simulink model "ASSIG2_v5"  (R2020a)
settings: Solver=FixedStepAuto  StartTime=0.0  StopTime=10.0  FixedStep=1e-3  RelTol=1e-3  EnableMultiTasking=on
undefined symbols (not defined in the file): A0, A1, D0, D1, D10, D11, D12, D13, D2, D3, D4, D5, D6, D7, D8, D9, magnitude, PTA0, PTA1, PTA2, PTB2, PTB23, PTB3, PTB9, PTC16, PTC17, PTC2, PTC3, PTC4, PTD0, PTD1, PTD2, PTD3
libraries: etargetslib x21, frdmk64flib x20
settings Model: ExtModeTrigDuration=5  Creator=Nour  LastModifiedBy=Khaled
settings OptimizationCC: EnhancedBackFolding=on  PassReuseOutputArgsAs=Individual arguments  ZeroExternalMemoryAtStartup=off  ZeroInternalMemoryAtStartup=off  MaxStackSize=64  OptimizeBlockOrder=speed  DifferentSizesBufferReuse=on  OptimizationCustomize=off  EfficientTunableParamExpr=on
settings DebuggingCC: ParameterTunabilityLossMsg=error  UnderSpecifiedDimensionMsg=error
settings HardwareCC: ProdBitPerPointer=32  ProdBitPerSizeT=32  ProdBitPerPtrDiffT=32  ProdLargestAtomicInteger=Long  ProdLargestAtomicFloat=Double  ProdWordSize=32  ProdHWDeviceType=ARM Compatible->ARM Cortex
settings SFSimCC: MATLABDynamicMemAlloc=off
settings RTWCC: SystemTargetFile=ert.tlc  HardwareBoard=NXP FRDM-K64F  TemplateMakefile=ert_default_tmf  Toolchain=GNU Tools for ARM Embedded Processors
settings CodeAppCC: ForceParamTrailComments=on  IgnoreCustomStorageClasses=off  OperatorAnnotations=on  SimulinkDataObjDesc=on  SFDataObjDesc=on  InsertBlockDesc=on

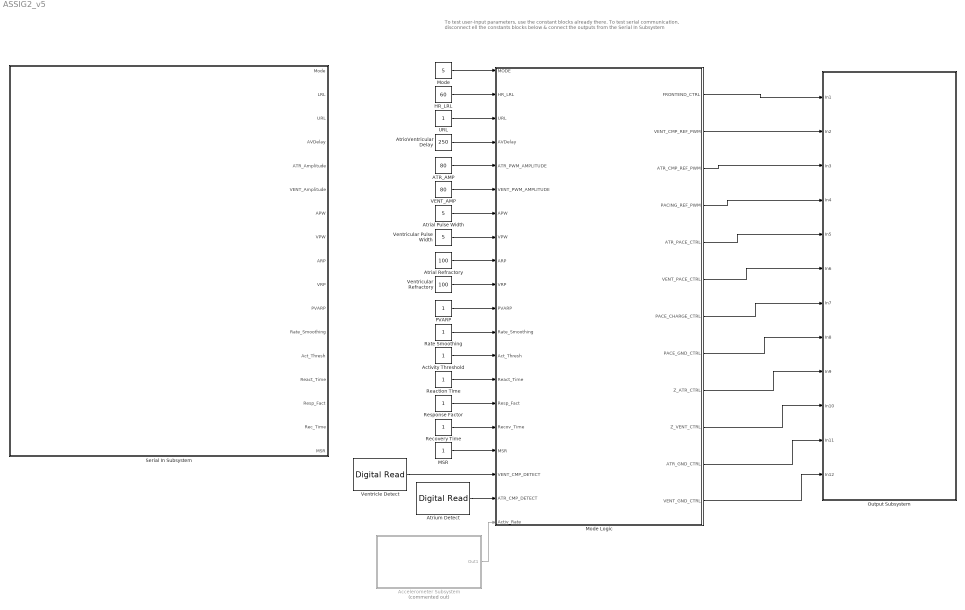
== system ASSIG2_v5 ==
  note: To test user-input parameters, use the constant blocks already there.
      | To test serial communication, disconnect ell the constants blocks below & connect the outputs from the Serial In Subsystem
  ATR_AMP : Constant  Value=80  OutDataTypeStr=uint8
  Accelerometer Subsystem : Subsystem  Commented=on
  Activity Threshold : Constant  OutDataTypeStr=single
  Atrial Pulse Width : Constant  Value=5  OutDataTypeStr=uint16
  Atrial Refractory : Constant  Value=100  OutDataTypeStr=uint16
  AtrioVentricular Delay : Constant  Value=250  OutDataTypeStr=uint16
  Atrium Detect : frdmk64flib/Digital Read  Whichpin=PTC16 (D0)  SampleTime=-1
  HR_LRL : Constant  Value=60  OutDataTypeStr=uint16
  MSR : Constant  OutDataTypeStr=uint16
  Mode : Constant  Value=5  OutDataTypeStr=uint8
  Mode Logic : Stateflow chart  TreatAsAtomicUnit=on
  Output Subsystem : Subsystem
  PVARP : Constant  OutDataTypeStr=uint16
  Rate Smoothing : Constant  OutDataTypeStr=uint8
  Reaction Time : Constant  OutDataTypeStr=uint16
  Recovery Time : Constant  OutDataTypeStr=uint16
  Response Factor : Constant  OutDataTypeStr=uint16
  Serial In Subsystem : Subsystem
  URL : Constant  OutDataTypeStr=uint8
  VENT_AMP : Constant  Value=80  OutDataTypeStr=uint8
  Ventricle Detect : frdmk64flib/Digital Read  Whichpin=PTC17 (D1)  SampleTime=-1
  Ventricular Pulse Width : Constant  Value=5  OutDataTypeStr=uint16
  Ventricular Refractory : Constant  Value=100  OutDataTypeStr=uint16
  wires:
  HR_LRL/1 -> Mode Logic/2(HR_LRL)
  Mode/1 -> Mode Logic/1(MODE)
  Atrial Refractory/1 -> Mode Logic/9(ARP)
  Ventricular Refractory/1 -> Mode Logic/10(VRP)
  Atrial Pulse Width/1 -> Mode Logic/7(APW)
  Ventricle Detect/1 -> Mode Logic/18(VENT_CMP_DETECT)
  Atrium Detect/1 -> Mode Logic/19(ATR_CMP_DETECT)
  Ventricular Pulse Width/1 -> Mode Logic/8(VPW)
  AtrioVentricular Delay/1 -> Mode Logic/4(AVDelay)
  MSR/1 -> Mode Logic/17(MSR)
  ATR_AMP/1 -> Mode Logic/5(ATR_PWM_AMPLITUDE)
  VENT_AMP/1 -> Mode Logic/6(VENT_PWM_AMPLITUDE)
  Mode Logic/1(FRONTEND_CTRL) -> Output Subsystem/1(In1)
  Mode Logic/2(VENT_CMP_REF_PWM) -> Output Subsystem/2(In2)
  Mode Logic/3(ATR_CMP_REF_PWM) -> Output Subsystem/3(In3)
  Mode Logic/4(PACING_REF_PWM) -> Output Subsystem/4(In4)
  Mode Logic/5(ATR_PACE_CTRL) -> Output Subsystem/5(In5)
  Mode Logic/6(VENT_PACE_CTRL) -> Output Subsystem/6(In6)
  Mode Logic/7(PACE_CHARGE_CTRL) -> Output Subsystem/7(In7)
  Mode Logic/8(PACE_GND_CTRL) -> Output Subsystem/8(In8)
  Mode Logic/9(Z_ATR_CTRL) -> Output Subsystem/9(In9)
  Mode Logic/10(Z_VENT_CTRL) -> Output Subsystem/10(In10)
  Mode Logic/11(ATR_GND_CTRL) -> Output Subsystem/11(In11)
  Mode Logic/12(VENT_GND_CTRL) -> Output Subsystem/12(In12)
  URL/1 -> Mode Logic/3(URL)
  PVARP/1 -> Mode Logic/11(PVARP)
  Recovery Time/1 -> Mode Logic/16(Recov_Time)
  Response Factor/1 -> Mode Logic/15(Resp_Fact)
  Reaction Time/1 -> Mode Logic/14(React_Time)
  Activity Threshold/1 -> Mode Logic/13(Act_Thresh)
  Rate Smoothing/1 -> Mode Logic/12(Rate_Smoothing)
  Accelerometer Subsystem/1(Out1) -> Mode Logic/20(Activ_Rate)

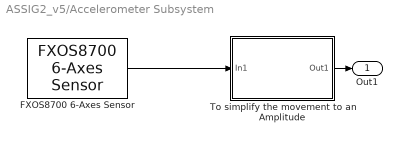
== system ASSIG2_v5/Accelerometer Subsystem ==
  FXOS8700 6-Axes Sensor : frdmk64flib/FXOS8700 6-Axes Sensor  Activesensor=Accelerometer only  ODR=800Hz  HybridODR=400Hz  Accelfullrange=-4g to +4g  SampleTime=-1
  To simplify the movement to an Amplitude : Subsystem
  Out1 : Outport
  wires:
  FXOS8700 6-Axes Sensor/1 -> To simplify the movement to an Amplitude/1(In1)
  To simplify the movement to an Amplitude/1(Out1) -> Out1/1

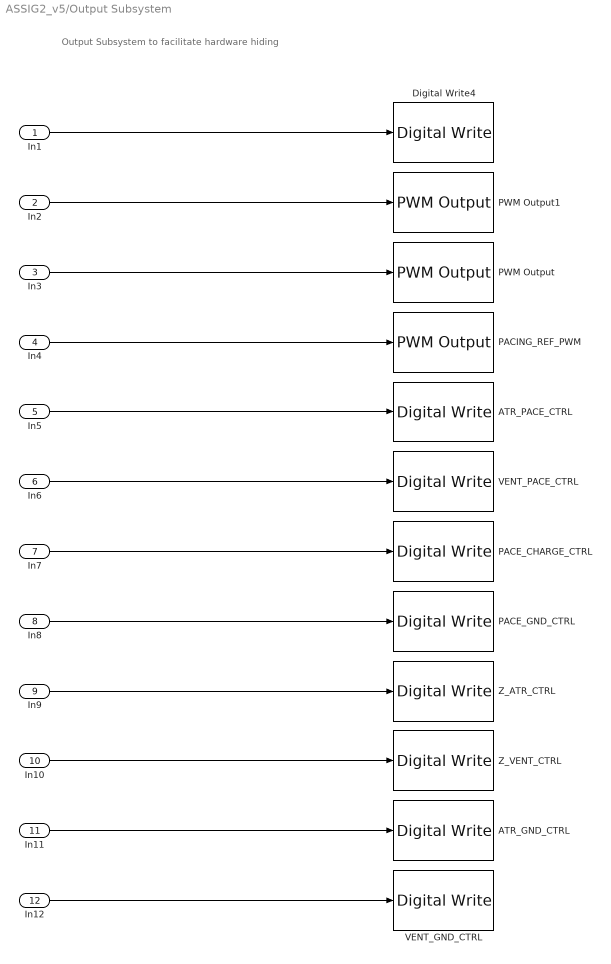
== system ASSIG2_v5/Output Subsystem ==
  note: Output Subsystem to facilitate hardware hiding
  In1 : Inport
  In2 : Inport  Port=2
  In3 : Inport  Port=3
  In4 : Inport  Port=4
  In5 : Inport  Port=5
  In6 : Inport  Port=6
  In7 : Inport  Port=7
  In8 : Inport  Port=8
  In9 : Inport  Port=9
  In10 : Inport  Port=10
  In11 : Inport  Port=11
  In12 : Inport  Port=12
  ATR_GND_CTRL : frdmk64flib/Digital Write  Whichpin=PTD2 (D11)
  ATR_PACE_CTRL : frdmk64flib/Digital Write  Whichpin=PTA0 (D8)
  Digital Write4 : frdmk64flib/Digital Write  Whichpin=PTD1 (D13)
  PACE_CHARGE_CTRL : frdmk64flib/Digital Write  Whichpin=PTB9 (D2)
  PACE_GND_CTRL : frdmk64flib/Digital Write  Whichpin=PTD0 (D10)
  PACING_REF_PWM : frdmk64flib/PWM Output  Whichpin=PTA2 (D5)  InitialFrequency=2000  InitialDutyCycle=80
  PWM Output : frdmk64flib/PWM Output  Whichpin=PTC2 (D6)  InitialFrequency=2000  InitialDutyCycle=20
  PWM Output1 : frdmk64flib/PWM Output  Whichpin=PTA1 (D3)  InitialFrequency=2000  InitialDutyCycle=20
  VENT_GND_CTRL : frdmk64flib/Digital Write  Whichpin=PTD3 (D12)
  VENT_PACE_CTRL : frdmk64flib/Digital Write  Whichpin=PTC4 (D9)
  Z_ATR_CTRL : frdmk64flib/Digital Write  Whichpin=PTB23 (D4)
  Z_VENT_CTRL : frdmk64flib/Digital Write  Whichpin=PTC3 (D7)
  wires:
  In7/1 -> PACE_CHARGE_CTRL/1
  In12/1 -> VENT_GND_CTRL/1
  In1/1 -> Digital Write4/1
  In4/1 -> PACING_REF_PWM/1
  In8/1 -> PACE_GND_CTRL/1
  In6/1 -> VENT_PACE_CTRL/1
  In9/1 -> Z_ATR_CTRL/1
  In10/1 -> Z_VENT_CTRL/1
  In11/1 -> ATR_GND_CTRL/1
  In2/1 -> PWM Output1/1
  In5/1 -> ATR_PACE_CTRL/1
  In3/1 -> PWM Output/1

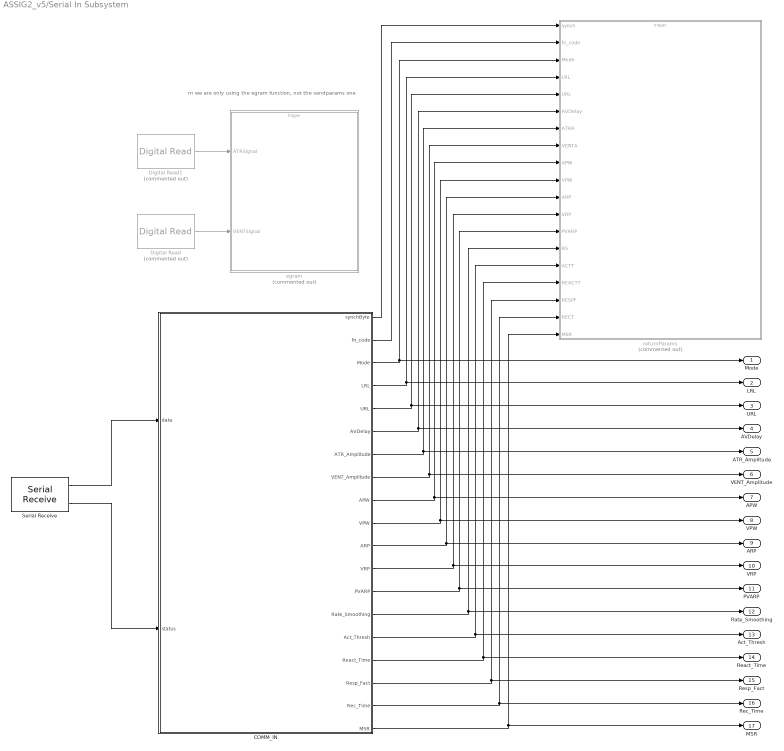
== system ASSIG2_v5/Serial In Subsystem ==
  note: rn we are only using the egram function, not the sendparams one
  COMM_IN : Stateflow chart  TreatAsAtomicUnit=on
  Digital Read : frdmk64flib/Digital Read  Commented=on  Whichpin=PTB3 (A1)  SampleTime=-1
  Digital Read1 : frdmk64flib/Digital Read  Commented=on  Whichpin=PTB2 (A0)  SampleTime=-1
  Serial Receive : frdmk64flib/Serial Receive  SCIModule=0  Baudrate=uint32(9600)  Parity=None  StopBits=1  HardwareFlowControl=None  ByteOrder=LittleEndian  DataType=uint8  DataLength=26  BlockingMode=off  OutputStatus=on  SampleTime=-1
  egram : Subsystem  Commented=on
  returnParams : Subsystem  Commented=on
  Mode : Outport
  LRL : Outport  Port=2
  URL : Outport  Port=3
  AVDelay : Outport  Port=4
  ATR_Amplitude : Outport  Port=5
  VENT_Amplitude : Outport  Port=6
  APW : Outport  Port=7
  VPW : Outport  Port=8
  ARP : Outport  Port=9
  VRP : Outport  Port=10
  PVARP : Outport  Port=11
  Rate_Smoothing : Outport  Port=12
  Act_Thresh : Outport  Port=13
  React_Time : Outport  Port=14
  Resp_Fact : Outport  Port=15
  Rec_Time : Outport  Port=16
  MSR : Outport  Port=17
  wires:
  COMM_IN/5(URL) -> returnParams/5(URL), URL/1
  COMM_IN/11(ARP) -> returnParams/11(ARP), ARP/1
  COMM_IN/6(AVDelay) -> returnParams/6(AVDelay), AVDelay/1
  Serial Receive/1 -> COMM_IN/1(data)
  COMM_IN/4(LRL) -> returnParams/4(LRL), LRL/1
  COMM_IN/10(VPW) -> returnParams/10(VPW), VPW/1
  Serial Receive/2 -> COMM_IN/2(status)
  COMM_IN/8(VENT_Amplitude) -> returnParams/8(VENTA), VENT_Amplitude/1
  COMM_IN/7(ATR_Amplitude) -> returnParams/7(ATRA), ATR_Amplitude/1
  COMM_IN/17(Resp_Fact) -> returnParams/17(RESPF), Resp_Fact/1
  COMM_IN/3(Mode) -> Mode/1, returnParams/3(Mode)
  COMM_IN/14(Rate_Smoothing) -> returnParams/14(RS), Rate_Smoothing/1
  COMM_IN/16(React_Time) -> returnParams/16(REACTT), React_Time/1
  COMM_IN/12(VRP) -> returnParams/12(VRP), VRP/1
  COMM_IN/9(APW) -> returnParams/9(APW), APW/1
  COMM_IN/18(Rec_Time) -> returnParams/18(RECT), Rec_Time/1
  COMM_IN/19(MSR) -> returnParams/19(MSR), MSR/1
  COMM_IN/15(Act_Thresh) -> returnParams/15(ACTT), Act_Thresh/1
  COMM_IN/13(PVARP) -> returnParams/13(PVARP), PVARP/1
  Digital Read1/1 -> egram/1(ATRSignal)
  Digital Read/1 -> egram/2(VENTSignal)
  COMM_IN/1(synchByte) -> returnParams/1(synch)
  COMM_IN/2(fn_code) -> returnParams/2(fn_code)

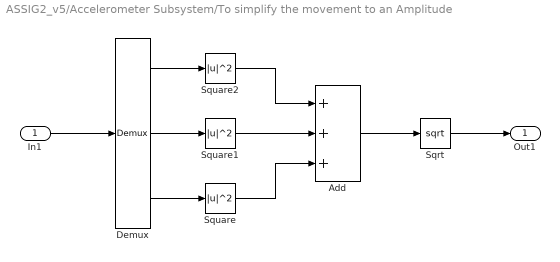
== system ASSIG2_v5/Accelerometer Subsystem/To simplify the movement to an Amplitude ==
  In1 : Inport
  Add : Sum  Inputs=+++
  Demux : Demux  Outputs=3
  Sqrt : Sqrt  OutputSignalType=real  OutDataTypeStr=single  IntermediateResultsDataTypeStr=double  SaturateOnIntegerOverflow=on
  Square : Math  Operator=magnitude^2  OutDataTypeStr=double  SaturateOnIntegerOverflow=on
  Square1 : Math  Operator=magnitude^2  OutDataTypeStr=double  SaturateOnIntegerOverflow=on
  Square2 : Math  Operator=magnitude^2  OutDataTypeStr=double  SaturateOnIntegerOverflow=on
  Out1 : Outport
  wires:
  In1/1 -> Demux/1
  Demux/3 -> Square/1
  Demux/2 -> Square1/1
  Demux/1 -> Square2/1
  Square2/1 -> Add/1
  Square1/1 -> Add/2
  Square/1 -> Add/3
  Add/1 -> Sqrt/1
  Sqrt/1 -> Out1/1

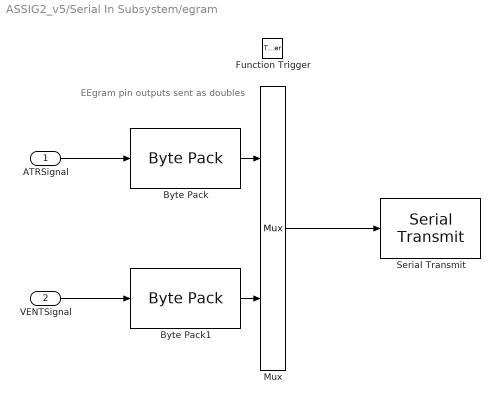
== system ASSIG2_v5/Serial In Subsystem/egram ==
  note: EEgram pin outputs sent as doubles
  ATRSignal : Inport
  VENTSignal : Inport  Port=2
  Function Trigger : TriggerPort  TriggerType=function-call  IsSimulinkFunction=on  FunctionName=eegram  VariantControl=Variant  PortDimensions=1
  Byte Pack : etargetslib/Byte Pack  datatypes={'double'}  byteAlign=1
  Byte Pack1 : etargetslib/Byte Pack  datatypes={'double'}  byteAlign=1
  Mux : Mux  Inputs=2
  Serial Transmit : frdmk64flib/Serial Transmit  SCIModule=0  Baudrate=uint32(9600)  Parity=None  StopBits=1  HardwareFlowControl=None  ByteOrder=LittleEndian  BlockingMode=on  OutputStatus=off
  wires:
  ATRSignal/1 -> Byte Pack/1
  Byte Pack1/1 -> Mux/2
  Byte Pack/1 -> Mux/1
  VENTSignal/1 -> Byte Pack1/1
  Mux/1 -> Serial Transmit/1

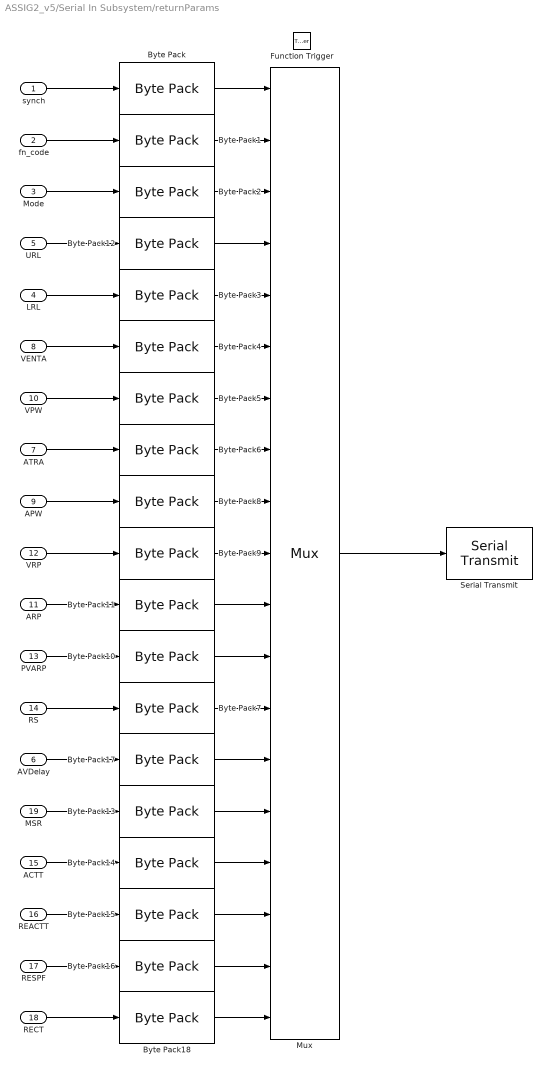
== system ASSIG2_v5/Serial In Subsystem/returnParams ==
  synch : Inport
  fn_code : Inport  Port=2
  Mode : Inport  Port=3
  LRL : Inport  Port=4
  URL : Inport  Port=5
  AVDelay : Inport  Port=6
  ATRA : Inport  Port=7
  VENTA : Inport  Port=8
  APW : Inport  Port=9
  VPW : Inport  Port=10
  ARP : Inport  Port=11
  VRP : Inport  Port=12
  PVARP : Inport  Port=13
  RS : Inport  Port=14
  ACTT : Inport  Port=15
  REACTT : Inport  Port=16
  RESPF : Inport  Port=17
  RECT : Inport  Port=18
  MSR : Inport  Port=19
  Function Trigger : TriggerPort  TriggerType=function-call  IsSimulinkFunction=on  FunctionName=returnParams  VariantControl=Variant  PortDimensions=1
  Byte Pack{,1..8,12..16,18} (15 alike) : etargetslib/Byte Pack  datatypes={'uint8'}  byteAlign=1
  Byte Pack{9..11,17} (4 alike) : etargetslib/Byte Pack  datatypes={'uint16'}  byteAlign=1
  Mux : Mux  Inputs=19
  Serial Transmit : frdmk64flib/Serial Transmit  SCIModule=0  Baudrate=uint32(9600)  Parity=None  StopBits=1  HardwareFlowControl=None  ByteOrder=LittleEndian  BlockingMode=on  OutputStatus=off
  wires:
  Byte Pack1/1 -> Mux/2
  Byte Pack/1 -> Mux/1
  Mux/1 -> Serial Transmit/1
  Byte Pack6/1 -> Mux/8
  Byte Pack2/1 -> Mux/3
  Byte Pack12/1 -> Mux/4
  Byte Pack3/1 -> Mux/5
  Byte Pack4/1 -> Mux/6
  Byte Pack5/1 -> Mux/7
  Byte Pack8/1 -> Mux/9
  Byte Pack11/1 -> Mux/11
  Byte Pack9/1 -> Mux/10
  Byte Pack10/1 -> Mux/12
  Byte Pack7/1 -> Mux/13
  Byte Pack16/1 -> Mux/18
  Byte Pack15/1 -> Mux/17
  Byte Pack14/1 -> Mux/16
  Byte Pack13/1 -> Mux/15
  Byte Pack17/1 -> Mux/14
  fn_code/1 -> Byte Pack1/1
  synch/1 -> Byte Pack/1
  Mode/1 -> Byte Pack2/1
  URL/1 -> Byte Pack12/1
  LRL/1 -> Byte Pack3/1
  VENTA/1 -> Byte Pack4/1
  VPW/1 -> Byte Pack5/1
  ATRA/1 -> Byte Pack6/1
  APW/1 -> Byte Pack8/1
  VRP/1 -> Byte Pack9/1
  ARP/1 -> Byte Pack11/1
  PVARP/1 -> Byte Pack10/1
  RS/1 -> Byte Pack7/1
  AVDelay/1 -> Byte Pack17/1
  MSR/1 -> Byte Pack13/1
  ACTT/1 -> Byte Pack14/1
  REACTT/1 -> Byte Pack15/1
  RESPF/1 -> Byte Pack16/1
  RECT/1 -> Byte Pack18/1
  Byte Pack18/1 -> Mux/19

== stateflow chart ASSIG2_v5/Serial In Subsystem/COMM_IN ==
  state SET_PARAM
    %% initial typecast of values through
    %% serial communication
    Mode = typecast(data(3), 'uint8');
    URL = typecast(data(4), 'uint8');
    LRL_t = typecast(data(5), 'uint8');
    VENT_Amplitude = typecast(data(6), 'uint8');
    VPW_t = typecast(data(7), 'uint8');
    ATR_Amplitude = typecast(data(8), 'uint8');
    APW_t = typecast(data(9), 'uint8');
    VRP = typecast(data(10:11), 'uint16');
    ARP = typecast(data(12:13), 'uint16');
    PVARP = typecast(data(14:15), 'uint16');
    Rate_Smoothing = typecast(data(16), 'uint8');
    AVDelay = typecast(data(17: 18), 'uint16');
    MSR_t = typecast(data(19), 'uint8');
    Act_Thresh = typecast(data(20:23), 'single');
    React_t = typecast(data(24), 'uint8');
    Resp_t = typecast(data(25), 'uint8');
    Rec_t = typecast(data(26), 'uint8');
    %% 2ndary typecast
    LRL  = uint16(LRL_t);
    VPW  = uint16(VPW_t);
    APW  = uint16(APW_t);
    MSR  = uint16(MSR_t);
    React_Time = uint16(React_t);
    Resp_Fact = uint16(Resp_t);
    Rec_Time = uint16(Rec_t);
  state INITIAL
    %% Setting initial, default values of parameters
    entry:
    Mode = 0;
    URL = 0;
    LRL = 0;
    VENT_Amplitude = 0;
    VPW = 0;
    ATR_Amplitude = 0;
    APW = 0;
    VRP = 0;
    ARP = 0;
    PVARP = 0;
    Rate_Smoothing = 0;
    AVDelay = 0;
    MSR = 0;
    Act_Thresh = 0;
    React_Time = 0;
    Resp_Fact = 0;
    Rec_Time = 0;
  state STANDBY
    %% Waiting for COM
    %% function code values;
    %% 55 -> set params
    %% 22 -> eegram
    %% 33 -> return params
    synchByte = typecast(data(1), 'uint8');
    fn_code = typecast(data(2), 'uint8');
  state EEGRAM
    entry:
    %%eegram();
  (junction 15) -> SET_PARAM [order 2] : [data(2) == hex2dec('55')]
  SET_PARAM -> STANDBY
  (default) -> INITIAL
  (junction 13) -> STANDBY [order 2]
  INITIAL -> STANDBY
  STANDBY -> (junction 13) : [status == 0]
  (junction 13) -> (junction 15) [order 1] : [data(1) == hex2dec('16')]
  (junction 15) -> EEGRAM [order 1] : [data(2) == hex2dec('22')]
  EEGRAM -> STANDBY
  data: synchByte output uint8; fn_code output uint8; data input uint8 size=[26;1]; status input uint8 size=[1;1]; Mode output uint8; LRL output uint16; URL output uint8; AVDelay output uint16; ATR_Amplitude output uint8; VENT_Amplitude output uint8; APW output uint16; VPW output uint16; ARP output uint16; VRP output uint16; PVARP output uint16; Rate_Smoothing output uint8; Act_Thresh output single; React_Time output uint16; Resp_Fact output uint16; Rec_Time output uint16; MSR output uint16; LRL_t local uint8; VPW_t local uint8; APW_t local uint8; MSR_t local uint8; React_t local uint8; Resp_t local uint8; Rec_t local uint8

== stateflow chart ASSIG2_v5/Mode Logic ==
  state AOO
    state CHARGE
      entry:
      ATR_PACE_CTRL = false;
      VENT_PACE_CTRL = false;
      PACING_REF_PWM = ATR_PWM_AMPLITUDE;
      PACE_CHARGE_CTRL = true;
      %Discharging Blocking Capacitor
      PACE_GND_CTRL = true;
      VENT_PACE_CTRL = false;
      Z_ATR_CTRL = false;
      Z_VENT_CTRL = false;
      %% ATR_PACE_CTRL = false;
      ATR_GND_CTRL = true;
      VENT_GND_CTRL = false;
    state PACE
      entry:
      PACE_CHARGE_CTRL = false;
      PACE_GND_CTRL = true;
      ATR_PACE_CTRL = true;
      ATR_GND_CTRL = false;
      Z_ATR_CTRL = false;
      Z_VENT_CTRL = false;
      VENT_GND_CTRL = false;
      VENT_PACE_CTRL = false;
    (default) -> AOO.CHARGE
    AOO.CHARGE -> AOO.PACE : [after((60000 / HR_LRL - APW), msec)]
    AOO.PACE -> AOO.CHARGE : [after(APW, msec)]
  state VOO
    state CHARGE
      %% Charge C22, Discharge C21
      entry:
      ATR_PACE_CTRL = false;
      VENT_PACE_CTRL = false;
      PACING_REF_PWM = VENT_PWM_AMPLITUDE;
      PACE_CHARGE_CTRL = true;
      %Dishcharging Blocking Capacitor
      PACE_GND_CTRL = true;
      Z_ATR_CTRL = false;
      Z_VENT_CTRL = false;
      ATR_GND_CTRL = false;
      VENT_GND_CTRL = true;
    state PACE
      entry:
      PACE_CHARGE_CTRL = false;
      PACE_GND_CTRL = true;
      ATR_PACE_CTRL = false;
      ATR_GND_CTRL = false;
      Z_ATR_CTRL = false;
      Z_VENT_CTRL = false;
      VENT_GND_CTRL = false;
      VENT_PACE_CTRL = true;
    (default) -> VOO.CHARGE
    VOO.CHARGE -> VOO.PACE : [after((60000 / HR_LRL - VPW), msec)]
    VOO.PACE -> VOO.CHARGE : [after(VPW, msec)]
  state Entry
    %% MODE Values:
    %% 1: AOO
    %% 2: VOO
    %% 3: AAI
    %% 4: VVI verify
    %% 5: DOO
    %% 6: AOOR
    %% 7: VOOR
    %% 8: AAIR
    %% 9:  VVIR
    %% 10: DOOR
    entry:
    ATR_CMP_REF_PWM = 80;
    VENT_CMP_REF_PWM = 20;
    delay = 0;
  state AAI
    state Charge
      entry:
      ATR_PACE_CTRL = false;
      VENT_PACE_CTRL = false;
      PACING_REF_PWM = ATR_PWM_AMPLITUDE;
      PACE_CHARGE_CTRL = true;
      %Discharging Blocking Capacitor
      PACE_GND_CTRL = true;
      VENT_PACE_CTRL = false;
      Z_ATR_CTRL = false;
      Z_VENT_CTRL = false;
      %% ATR_PACE_CTRL = false;
      ATR_GND_CTRL = true;
      VENT_GND_CTRL = false;
      FRONTEND_CTRL = true;
    state Pace
      entry:
      PACE_CHARGE_CTRL = false;
      PACE_GND_CTRL = true;
      ATR_PACE_CTRL = true;
      ATR_GND_CTRL = false;
      Z_ATR_CTRL = false;
      Z_VENT_CTRL = false;
      VENT_GND_CTRL = false;
      VENT_PACE_CTRL = false;
      %% FRONTEND_CTRL = true;
    state Refractor
      entry:
      ATR_PACE_CTRL = false;
      VENT_PACE_CTRL = false;
      PACING_REF_PWM = ATR_PWM_AMPLITUDE;
      PACE_CHARGE_CTRL = true;
      %Discharging Blocking Capacitor
      PACE_GND_CTRL = true;
      VENT_PACE_CTRL = false;
      Z_ATR_CTRL = false;
      Z_VENT_CTRL = false;
      %% ATR_PACE_CTRL = false;
      ATR_GND_CTRL = true;
      VENT_GND_CTRL = false;
      %% FRONTEND_CTRL = true;
    (default) -> AAI.Charge
    AAI.Charge -> AAI.Pace [order 1] : [after((60000 / HR_LRL - ARP - delay), msec)]
    AAI.Charge -> AAI.Refractor [order 2] : [ATR_CMP_DETECT == true]{delay = 0}
    AAI.Refractor -> AAI.Charge : [after(ARP, msec)]
    AAI.Pace -> AAI.Refractor : [after(APW, msec)]{delay = APW}
  state DOOR
    state ATRCharge
      entry:
      ATR_PACE_CTRL = false;
      VENT_PACE_CTRL = false;
      PACING_REF_PWM = ATR_PWM_AMPLITUDE;
      PACE_CHARGE_CTRL = true;
      %Discharging Blocking Capacitor
      PACE_GND_CTRL = true;
      VENT_PACE_CTRL = false;
      Z_ATR_CTRL = false;
      Z_VENT_CTRL = false;
      %% ATR_PACE_CTRL = false;
      ATR_GND_CTRL = true;
      VENT_GND_CTRL = false;
      state ENTRY_STATE
        entry:
        prev_HR_LRL = HR_LRLR;
        ReqI_HR_LRL = (MSR - HR_LRL) * (Resp_Fact / 16) + HR_LRL;
        %% Final_dHR is just HR_LRL
        ReqD_HR_LRL = HR_LRL;
      state Increment_HR
        entry:
        deltaI_HR = ReqI_HR_LRL - HR_LRL;
        HR_LRLR = floor(prev_HR_LRL + (deltaI_HR * 60)/(HR_LRL * React_Time));
      state Maintain_HR
        entry:
        HR_LRLR = prev_HR_LRL;
      state Decrement_HR
        entry:
        deltaD_HR = (MSR + prev_HR_LRL) / 2 - ReqD_HR_LRL;
        HR_LRLR = floor(prev_HR_LRL - (deltaD_HR * 60) / (HR_LRL * Recov_Time))
      (default) -> DOOR.ATRCharge.ENTRY_STATE
      DOOR.ATRCharge.ENTRY_STATE -> (junction 246) [order 2] : [Activ_Rate < Act_Thresh]
      DOOR.ATRCharge.ENTRY_STATE -> (junction 253) [order 1] : [Activ_Rate >= Act_Thresh]
      (junction 253) -> DOOR.ATRCharge.Maintain_HR [order 2] : [ReqI_HR_LRL <= prev_HR_LRL]
      (junction 253) -> DOOR.ATRCharge.Increment_HR [order 1] : [ReqI_HR_LRL > prev_HR_LRL]
      (junction 246) -> DOOR.ATRCharge.Maintain_HR [order 1] : [prev_HR_LRL <= ReqD_HR_LRL]
      (junction 246) -> DOOR.ATRCharge.Decrement_HR [order 2] : [prev_HR_LRL > ReqD_HR_LRL]
    state ATRPace
      entry:
      entry:
      PACE_CHARGE_CTRL = false;
      PACE_GND_CTRL = true;
      ATR_PACE_CTRL = true;
      ATR_GND_CTRL = false;
      Z_ATR_CTRL = false;
      Z_VENT_CTRL = false;
      VENT_GND_CTRL = false;
      VENT_PACE_CTRL = false;
    state VENTCharge
      %% Charge C22, Discharge C21
      entry:
      ATR_PACE_CTRL = false;
      VENT_PACE_CTRL = false;
      PACING_REF_PWM = VENT_PWM_AMPLITUDE;
      PACE_CHARGE_CTRL = true;
      %Dishcharging Blocking Capacitor
      PACE_GND_CTRL = true;
      Z_ATR_CTRL = false;
      Z_VENT_CTRL = false;
      ATR_GND_CTRL = false;
      VENT_GND_CTRL = true;
    state VentPace
      entry:
      PACE_CHARGE_CTRL = false;
      PACE_GND_CTRL = true;
      ATR_PACE_CTRL = false;
      ATR_GND_CTRL = false;
      Z_ATR_CTRL = false;
      Z_VENT_CTRL = false;
      VENT_GND_CTRL = false;
      VENT_PACE_CTRL = true;
    (default) -> DOOR.ATRCharge : {HR_LRLR = HR_LRL}
    DOOR.ATRCharge -> DOOR.ATRPace : [after((60000 / HR_LRLR - AVDelay - APW - VPW), msec)]
    DOOR.ATRPace -> DOOR.VENTCharge : [after(APW, msec)]
    DOOR.VentPace -> DOOR.ATRCharge : [after(VPW, msec)]
    DOOR.VENTCharge -> DOOR.VentPace : [after(AVDelay, msec)]
  state VVI
    state Charge
      %% Charge C22, Discharge C21
      entry:
      ATR_PACE_CTRL = false;
      VENT_PACE_CTRL = false;
      PACING_REF_PWM = VENT_PWM_AMPLITUDE;
      PACE_CHARGE_CTRL = true;
      %Dishcharging Blocking Capacitor
      PACE_GND_CTRL = true;
      Z_ATR_CTRL = false;
      Z_VENT_CTRL = false;
      ATR_GND_CTRL = false;
      VENT_GND_CTRL = true;
      FRONTEND_CTRL = true;
    state Pace
      entry:
      PACE_CHARGE_CTRL = false;
      PACE_GND_CTRL = true;
      ATR_PACE_CTRL = false;
      ATR_GND_CTRL = false;
      Z_ATR_CTRL = false;
      Z_VENT_CTRL = false;
      VENT_GND_CTRL = false;
      VENT_PACE_CTRL = true;
      %% FRONTEND_CTRL = true;
    state Refractor
      %% Charge C22, Discharge C21
      entry:
      ATR_PACE_CTRL = false;
      VENT_PACE_CTRL = false;
      PACING_REF_PWM = VENT_PWM_AMPLITUDE;
      PACE_CHARGE_CTRL = true;
      %Dishcharging Blocking Capacitor
      PACE_GND_CTRL = true;
      Z_ATR_CTRL = false;
      Z_VENT_CTRL = false;
      ATR_GND_CTRL = false;
      VENT_GND_CTRL = true;
      %% FRONTEND_CTRL = true;
    (default) -> VVI.Charge
    VVI.Charge -> VVI.Pace [order 1] : [after((60000 / HR_LRL - VRP - delay), msec)]
    VVI.Charge -> VVI.Refractor [order 2] : [VENT_CMP_DETECT == true]{delay = 0}
    VVI.Refractor -> VVI.Charge : [after(VRP, msec)]
    VVI.Pace -> VVI.Refractor : [after(VPW, msec)]{delay = VPW}
  state VVIR
    state Charge
      %% Charge C22, Discharge C21
      entry:
      ATR_PACE_CTRL = false;
      VENT_PACE_CTRL = false;
      PACING_REF_PWM = VENT_PWM_AMPLITUDE;
      PACE_CHARGE_CTRL = true;
      %Dishcharging Blocking Capacitor
      PACE_GND_CTRL = true;
      Z_ATR_CTRL = false;
      Z_VENT_CTRL = false;
      ATR_GND_CTRL = false;
      VENT_GND_CTRL = true;
      FRONTEND_CTRL = true;
      state ENTRY_STATE
        entry:
        prev_HR_LRL = HR_LRLR;
        ReqI_HR_LRL = (MSR - HR_LRL) * (Resp_Fact / 16) + HR_LRL;
        %% Final_dHR is just HR_LRL
        ReqD_HR_LRL = HR_LRL;
      state Increment_HR
        entry:
        deltaI_HR = ReqI_HR_LRL - HR_LRL;
        HR_LRLR = floor(prev_HR_LRL + (deltaI_HR * 60)/(HR_LRL * React_Time));
      state Maintain_HR
        entry:
        HR_LRLR = prev_HR_LRL;
      state Decrement_HR
        entry:
        deltaD_HR = (MSR + prev_HR_LRL) / 2 - ReqD_HR_LRL;
        HR_LRLR = floor(prev_HR_LRL - (deltaD_HR * 60) / (HR_LRL * Recov_Time))
      (default) -> VVIR.Charge.ENTRY_STATE
      VVIR.Charge.ENTRY_STATE -> (junction 233) [order 2] : [Activ_Rate < Act_Thresh]
      VVIR.Charge.ENTRY_STATE -> (junction 240) [order 1] : [Activ_Rate >= Act_Thresh]
      (junction 240) -> VVIR.Charge.Maintain_HR [order 2] : [ReqI_HR_LRL <= prev_HR_LRL]
      (junction 240) -> VVIR.Charge.Increment_HR [order 1] : [ReqI_HR_LRL > prev_HR_LRL]
      (junction 233) -> VVIR.Charge.Maintain_HR [order 1] : [prev_HR_LRL <= ReqD_HR_LRL]
      (junction 233) -> VVIR.Charge.Decrement_HR [order 2] : [prev_HR_LRL > ReqD_HR_LRL]
    state Pace
      entry:
      PACE_CHARGE_CTRL = false;
      PACE_GND_CTRL = true;
      ATR_PACE_CTRL = false;
      ATR_GND_CTRL = false;
      Z_ATR_CTRL = false;
      Z_VENT_CTRL = false;
      VENT_GND_CTRL = false;
      VENT_PACE_CTRL = true;
      %% FRONTEND_CTRL = true;
    state Refractor
      %% Charge C22, Discharge C21
      entry:
      ATR_PACE_CTRL = false;
      VENT_PACE_CTRL = false;
      PACING_REF_PWM = VENT_PWM_AMPLITUDE;
      PACE_CHARGE_CTRL = true;
      %Dishcharging Blocking Capacitor
      PACE_GND_CTRL = true;
      Z_ATR_CTRL = false;
      Z_VENT_CTRL = false;
      ATR_GND_CTRL = false;
      VENT_GND_CTRL = true;
      %% FRONTEND_CTRL = true;
    (default) -> VVIR.Charge : {HR_LRLR = HR_LRL}
    VVIR.Charge -> VVIR.Refractor [order 2] : [VENT_CMP_DETECT == true]{delay = 0}
    VVIR.Charge -> VVIR.Pace [order 1] : [after((60000 / HR_LRLR - VRP - delay), msec)]
    VVIR.Refractor -> VVIR.Charge : [after(VRP, msec)]
    VVIR.Pace -> VVIR.Refractor : [after(VPW, msec)]{delay = VPW}
  state AAIR
    state Charge
      entry:
      ATR_PACE_CTRL = false;
      VENT_PACE_CTRL = false;
      PACING_REF_PWM = ATR_PWM_AMPLITUDE;
      PACE_CHARGE_CTRL = true;
      %Discharging Blocking Capacitor
      PACE_GND_CTRL = true;
      VENT_PACE_CTRL = false;
      Z_ATR_CTRL = false;
      Z_VENT_CTRL = false;
      %% ATR_PACE_CTRL = false;
      ATR_GND_CTRL = true;
      VENT_GND_CTRL = false;
      FRONTEND_CTRL = true;
      state ENTRY_STATE
        entry:
        prev_HR_LRL = HR_LRLR;
        ReqI_HR_LRL = (MSR - HR_LRL) * (Resp_Fact / 16) + HR_LRL;
        %% Final_dHR is just HR_LRL
        ReqD_HR_LRL = HR_LRL;
      state Increment_HR
        entry:
        deltaI_HR = ReqI_HR_LRL - HR_LRL;
        HR_LRLR = floor(prev_HR_LRL + (deltaI_HR * 60)/(HR_LRL * React_Time));
      state Maintain_HR
        entry:
        HR_LRLR = prev_HR_LRL;
      state Decrement_HR
        entry:
        deltaD_HR = (MSR + prev_HR_LRL) / 2 - ReqD_HR_LRL;
        HR_LRLR = floor(prev_HR_LRL - (deltaD_HR * 60) / (HR_LRL * Recov_Time))
      (default) -> AAIR.Charge.ENTRY_STATE
      AAIR.Charge.ENTRY_STATE -> (junction 220) [order 2] : [Activ_Rate < Act_Thresh]
      AAIR.Charge.ENTRY_STATE -> (junction 227) [order 1] : [Activ_Rate >= Act_Thresh]
      (junction 227) -> AAIR.Charge.Maintain_HR [order 2] : [ReqI_HR_LRL <= prev_HR_LRL]
      (junction 227) -> AAIR.Charge.Increment_HR [order 1] : [ReqI_HR_LRL > prev_HR_LRL]
      (junction 220) -> AAIR.Charge.Maintain_HR [order 1] : [prev_HR_LRL <= ReqD_HR_LRL]
      (junction 220) -> AAIR.Charge.Decrement_HR [order 2] : [prev_HR_LRL > ReqD_HR_LRL]
    state Pace
      entry:
      PACE_CHARGE_CTRL = false;
      PACE_GND_CTRL = true;
      ATR_PACE_CTRL = true;
      ATR_GND_CTRL = false;
      Z_ATR_CTRL = false;
      Z_VENT_CTRL = false;
      VENT_GND_CTRL = false;
      VENT_PACE_CTRL = false;
      %% FRONTEND_CTRL = true;
    state Refractor
      entry:
      ATR_PACE_CTRL = false;
      VENT_PACE_CTRL = false;
      PACING_REF_PWM = ATR_PWM_AMPLITUDE;
      PACE_CHARGE_CTRL = true;
      %Discharging Blocking Capacitor
      PACE_GND_CTRL = true;
      VENT_PACE_CTRL = false;
      Z_ATR_CTRL = false;
      Z_VENT_CTRL = false;
      %% ATR_PACE_CTRL = false;
      ATR_GND_CTRL = true;
      VENT_GND_CTRL = false;
      %% FRONTEND_CTRL = true;
    (default) -> AAIR.Charge : {HR_LRLR = HR_LRL}
    AAIR.Charge -> AAIR.Pace [order 1] : [after((60000 / HR_LRLR - ARP - delay), msec)]
    AAIR.Charge -> AAIR.Refractor [order 2] : [ATR_CMP_DETECT == true]{delay = 0}
    AAIR.Refractor -> AAIR.Charge : [after(ARP, msec)]
    AAIR.Pace -> AAIR.Refractor : [after(APW, msec)]{delay = APW}
  state DOO
    state ATRCharge
      entry:
      ATR_PACE_CTRL = false;
      VENT_PACE_CTRL = false;
      PACING_REF_PWM = ATR_PWM_AMPLITUDE;
      PACE_CHARGE_CTRL = true;
      %Discharging Blocking Capacitor
      PACE_GND_CTRL = true;
      VENT_PACE_CTRL = false;
      Z_ATR_CTRL = false;
      Z_VENT_CTRL = false;
      %% ATR_PACE_CTRL = false;
      ATR_GND_CTRL = true;
      VENT_GND_CTRL = false;
    state ATRPace
      entry:
      entry:
      PACE_CHARGE_CTRL = false;
      PACE_GND_CTRL = true;
      ATR_PACE_CTRL = true;
      ATR_GND_CTRL = false;
      Z_ATR_CTRL = false;
      Z_VENT_CTRL = false;
      VENT_GND_CTRL = false;
      VENT_PACE_CTRL = false;
    state VENTCharge
      %% Charge C22, Discharge C21
      entry:
      ATR_PACE_CTRL = false;
      VENT_PACE_CTRL = false;
      PACING_REF_PWM = VENT_PWM_AMPLITUDE;
      PACE_CHARGE_CTRL = true;
      %Dishcharging Blocking Capacitor
      PACE_GND_CTRL = true;
      Z_ATR_CTRL = false;
      Z_VENT_CTRL = false;
      ATR_GND_CTRL = false;
      VENT_GND_CTRL = true;
    state VentPace
      entry:
      PACE_CHARGE_CTRL = false;
      PACE_GND_CTRL = true;
      ATR_PACE_CTRL = false;
      ATR_GND_CTRL = false;
      Z_ATR_CTRL = false;
      Z_VENT_CTRL = false;
      VENT_GND_CTRL = false;
      VENT_PACE_CTRL = true;
    (default) -> DOO.ATRCharge
    DOO.ATRCharge -> DOO.ATRPace : [after((60000 / HR_LRL - AVDelay - APW - VPW), msec)]
    DOO.ATRPace -> DOO.VENTCharge : [after(APW, msec)]
    DOO.VentPace -> DOO.ATRCharge : [after(VPW, msec)]
    DOO.VENTCharge -> DOO.VentPace : [after(AVDelay, msec)]
  state VOOR
    state CHARGE
      %% Charge C22, Discharge C21
      entry:
      ATR_PACE_CTRL = false;
      VENT_PACE_CTRL = false;
      PACING_REF_PWM = VENT_PWM_AMPLITUDE;
      PACE_CHARGE_CTRL = true;
      %Dishcharging Blocking Capacitor
      PACE_GND_CTRL = true;
      Z_ATR_CTRL = false;
      Z_VENT_CTRL = false;
      ATR_GND_CTRL = false;
      VENT_GND_CTRL = true;
      state ENTRY_STATE
        entry:
        prev_HR_LRL = HR_LRLR;
        ReqI_HR_LRL = (MSR - HR_LRL) * (Resp_Fact / 16) + HR_LRL;
        %% Final_dHR is just HR_LRL
        ReqD_HR_LRL = HR_LRL;
      state Increment_HR
        entry:
        deltaI_HR = ReqI_HR_LRL - HR_LRL;
        HR_LRLR = floor(prev_HR_LRL + (deltaI_HR * 60)/(HR_LRL * React_Time));
      state Maintain_HR
        entry:
        HR_LRLR = prev_HR_LRL;
      state Decrement_HR
        entry:
        deltaD_HR = (MSR + prev_HR_LRL) / 2 - ReqD_HR_LRL;
        HR_LRLR = floor(prev_HR_LRL - (deltaD_HR * 60) / (HR_LRL * Recov_Time))
      (default) -> VOOR.CHARGE.ENTRY_STATE
      VOOR.CHARGE.ENTRY_STATE -> (junction 185) [order 2] : [Activ_Rate < Act_Thresh]
      VOOR.CHARGE.ENTRY_STATE -> (junction 181) [order 1] : [Activ_Rate >= Act_Thresh]
      (junction 181) -> VOOR.CHARGE.Maintain_HR [order 2] : [ReqI_HR_LRL <= prev_HR_LRL]
      (junction 181) -> VOOR.CHARGE.Increment_HR [order 1] : [ReqI_HR_LRL > prev_HR_LRL]
      (junction 185) -> VOOR.CHARGE.Maintain_HR [order 1] : [prev_HR_LRL <= ReqD_HR_LRL]
      (junction 185) -> VOOR.CHARGE.Decrement_HR [order 2] : [prev_HR_LRL > ReqD_HR_LRL]
    state PACE
      entry:
      PACE_CHARGE_CTRL = false;
      PACE_GND_CTRL = true;
      ATR_PACE_CTRL = false;
      ATR_GND_CTRL = false;
      Z_ATR_CTRL = false;
      Z_VENT_CTRL = false;
      VENT_GND_CTRL = false;
      VENT_PACE_CTRL = true;
    (default) -> VOOR.CHARGE : {HR_LRLR = HR_LRL}
    VOOR.CHARGE -> VOOR.PACE : [after((60000 / HR_LRLR - VPW), msec)]
    VOOR.PACE -> VOOR.CHARGE : [after(VPW, msec)]
  state AOOR
    state CHARGE
      entry:
      ATR_PACE_CTRL = false;
      VENT_PACE_CTRL = false;
      PACING_REF_PWM = ATR_PWM_AMPLITUDE;
      PACE_CHARGE_CTRL = true;
      %Discharging Blocking Capacitor
      PACE_GND_CTRL = true;
      VENT_PACE_CTRL = false;
      Z_ATR_CTRL = false;
      Z_VENT_CTRL = false;
      %% ATR_PACE_CTRL = false;
      ATR_GND_CTRL = true;
      VENT_GND_CTRL = false;
      state ENTRY_STATE
        entry:
        prev_HR_LRL = HR_LRLR;
        ReqI_HR_LRL = (MSR - HR_LRL) * (Resp_Fact / 16) + HR_LRL;
        %% Final_dHR is just HR_LRL
        ReqD_HR_LRL = HR_LRL;
      state Increment_HR
        entry:
        deltaI_HR = ReqI_HR_LRL - HR_LRL;
        HR_LRLR = floor(prev_HR_LRL + (deltaI_HR * 60)/(HR_LRL * React_Time));
      state Maintain_HR
        entry:
        HR_LRLR = prev_HR_LRL;
      state Decrement_HR
        entry:
        deltaD_HR = (MSR + prev_HR_LRL) / 2 - ReqD_HR_LRL;
        HR_LRLR = floor(prev_HR_LRL - (deltaD_HR * 60) / (HR_LRL * Recov_Time))
      (default) -> AOOR.CHARGE.ENTRY_STATE
      AOOR.CHARGE.ENTRY_STATE -> (junction 155) [order 2] : [Activ_Rate < Act_Thresh]
      AOOR.CHARGE.ENTRY_STATE -> (junction 151) [order 1] : [Activ_Rate >= Act_Thresh]
      (junction 151) -> AOOR.CHARGE.Maintain_HR [order 2] : [ReqI_HR_LRL <= prev_HR_LRL]
      (junction 151) -> AOOR.CHARGE.Increment_HR [order 1] : [ReqI_HR_LRL > prev_HR_LRL]
      (junction 155) -> AOOR.CHARGE.Maintain_HR [order 1] : [prev_HR_LRL <= ReqD_HR_LRL]
      (junction 155) -> AOOR.CHARGE.Decrement_HR [order 2] : [prev_HR_LRL > ReqD_HR_LRL]
    state PACE
      entry:
      PACE_CHARGE_CTRL = false;
      PACE_GND_CTRL = true;
      ATR_PACE_CTRL = true;
      ATR_GND_CTRL = false;
      Z_ATR_CTRL = false;
      Z_VENT_CTRL = false;
      VENT_GND_CTRL = false;
      VENT_PACE_CTRL = false;
    (default) -> AOOR.CHARGE : {HR_LRLR = HR_LRL}
    AOOR.CHARGE -> AOOR.PACE : [after((60000 / HR_LRLR - APW), msec)]
    AOOR.PACE -> AOOR.CHARGE : [after(APW, msec)]
  Entry -> AOO [order 1] : [MODE == 1]
  AOO -> Entry : [MODE ~= 1]
  Entry -> VOO [order 2] : [MODE == 2]
  VOO -> Entry : [MODE ~= 2]
  (default) -> Entry
  Entry -> AAI [order 4] : [MODE == 3]
  Entry -> DOOR [order 10] : [MODE == 10]
  AAI -> Entry : [MODE ~= 3]
  DOOR -> Entry : [MODE ~= 10]
  Entry -> VVI [order 5] : [MODE == 4]
  Entry -> VVIR [order 9] : [MODE == 9]
  VVI -> Entry : [MODE ~= 4]
  VVIR -> Entry : [MODE ~= 9]
  Entry -> AAIR [order 8] : [MODE == 8]
  Entry -> DOO [order 3] : [MODE == 5]
  AAIR -> Entry : [MODE ~= 8]
  DOO -> Entry : [MODE ~= 5]
  VOOR -> Entry : [MODE ~= 7]
  Entry -> VOOR [order 7] : [MODE == 7]
  Entry -> AOOR [order 6] : [MODE == 6]
  AOOR -> Entry : [MODE ~= 6]
  data: MODE input uint8; FRONTEND_CTRL output boolean; delay local uint16; HR_LRL input uint16; URL input uint8; AVDelay input uint16; ATR_PWM_AMPLITUDE input uint8; VENT_PWM_AMPLITUDE input uint8; APW input uint16; VPW input uint16; VENT_CMP_REF_PWM output uint16; ATR_CMP_REF_PWM output uint16; ARP input uint16; VRP input uint16; PVARP input uint16; Rate_Smoothing input uint8; Act_Thresh input single; React_Time input uint16; Resp_Fact input uint16; Recov_Time input uint16; MSR input uint16; VENT_CMP_DETECT input boolean; ATR_CMP_DETECT input boolean; PACING_REF_PWM output uint8; ATR_PACE_CTRL output boolean; VENT_PACE_CTRL output boolean; PACE_CHARGE_CTRL output boolean; PACE_GND_CTRL output boolean; Z_ATR_CTRL output boolean; Z_VENT_CTRL output boolean; ATR_GND_CTRL output boolean; VENT_GND_CTRL output boolean; HR_LRLR local uint16; Activ_Rate input single; prev_HR_LRL local uint16; ReqI_HR_LRL local uint16; deltaI_HR local uint16; ReqD_HR_LRL local uint16; deltaD_HR local uint16
